simulink model "ColorCodingExample"  (Simulink 7.5)
settings: Solver=FixedStepDiscrete  StartTime=0.0  StopTime=0  FixedStep=0.01  RelTol=1e-3
PostLoadFcn:
  | Workspace_Variable = 1;
InitFcn:
  | ViewValues(1);
undefined symbols (not defined in the file or in its folder): C
libraries: CSA_Library x1
settings Model: Creator=healypa  LastModifiedBy=sufanmi
settings OptimizationCC: InlineInvariantSignals=on  InitFltsAndDblsToZero=on
settings DebuggingCC: SaveWithDisabledLinksMsg=none  SaveWithParameterizedLinksMsg=none  SignalResolutionControl=TryResolveAllWithWarning  MultiTaskDSMMsg=warning  MultiTaskCondExecSysMsg=none  StrictBusMsg=None
settings RTWCC: IncludeERTFirstTime=on
settings GRTTargetCC: TargetFcnLib=ansi_tfl_tmw.mat

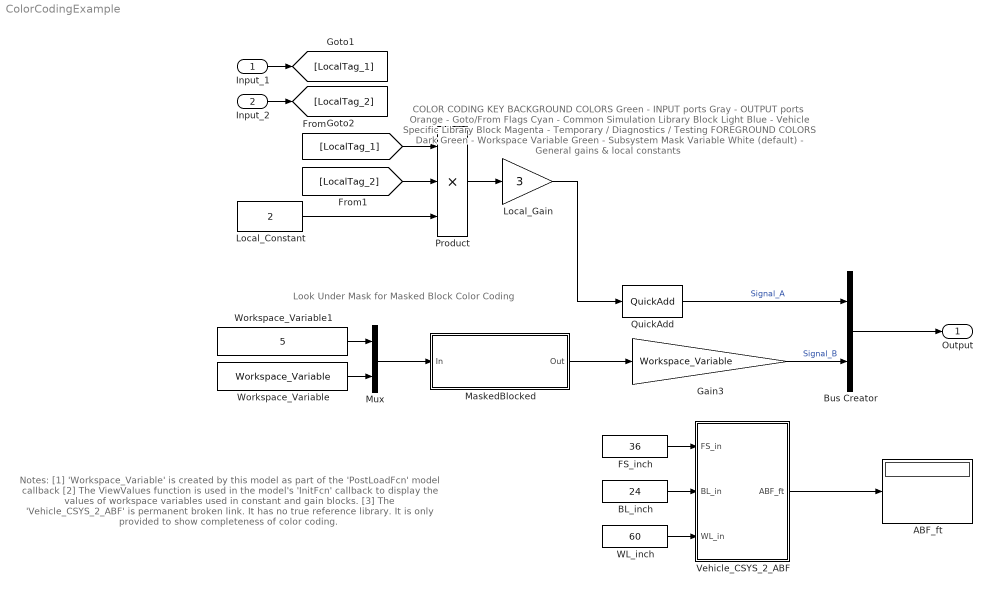
== system ColorCodingExample ==
  note: COLOR CODING KEY
      |
      | BACKGROUND COLORS
      | Green                 - INPUT ports
      | Gray                   - OUTPUT ports
      | Orange               - Goto/From Flags
      | Cyan                   - Common Simulation Library Block
      | Light Blue          - Vehicle Specific Library Block
      | Magenta             - Temporary / Diagnostics / Testing
      |
      | FOREGROUND COLORS
      | Dark Green       - Workspace Variable
      | Green                 - Subsystem Mask Variable
      | White (default) - General gains & local constants
  note: Look Under Mask for
      | Masked Block
      | Color Coding
  note: Notes:
      |
      | [1]  'Workspace_Variable' is created by this
      |        model as part of the 'PostLoadFcn' model callback
      |
      | [2]  The ViewValues function is used in the model's
      |        'InitFcn' callback to display the values of workspace
      |        variables used in constant and gain blocks.
      |
      | [3] The 'Vehicle_CSYS_2_ABF' is permanent broken
      |        link.  It has no true reference library.  It is only
      |        provided to show completeness of color coding.
  Input_1 : Inport  OutDataType=sfix(16)  OutScaling=2^0
  Input_2 : Inport  Port=2  OutDataType=sfix(16)  OutScaling=2^0
  ABF_ft : Display
  BL_inch : Constant  Value=24  OutDataType=sfix(16)  OutScaling=2^0
  Bus Creator : BusCreator  Inputs=2
  FS_inch : Constant  Value=36  OutDataType=sfix(16)  OutScaling=2^0
  Gain3 : Gain  Tag=5  Gain=Workspace_Variable  ParameterDataType=sfix(16)  ParameterScaling=2^0  OutDataType=sfix(16)  OutScaling=2^0
      settings: AttributesFormatString=value: 1
  Local_Constant : Constant  Value=2  OutDataType=sfix(16)  OutScaling=2^0
  Local_Gain : Gain  Gain=3  ParameterDataType=sfix(16)  ParameterScaling=2^0  OutDataType=sfix(16)  OutScaling=2^0
  MaskedBlocked : Subsystem  mask{Mask_Variable=0}
      mask prompts: Mask_Variable "Masked Variable Value"
      mask Display:
      | disp('Masked Block')
      | port_label('input',1,'In');
      | port_label('output',1,'Out');
  Mux : Mux  Inputs=2
  Product : Product  Inputs=3  OutDataType=sfix(16)  OutScaling=2^0  RndMeth=Zero
  QuickAdd : CSA_Library/Utilities/QuickAdd  SystemSampleTime=-1  mskValue=1
  Vehicle_CSYS_2_ABF : Subsystem  AncestorBlock=CSA_Library/Utilities/Vehicle_CSYS_2_ABF
  WL_inch : Constant  Value=60  OutDataType=sfix(16)  OutScaling=2^0
  Workspace_Variable : Constant  Tag=5  Value=Workspace_Variable  OutDataType=sfix(16)  OutScaling=2^0
      settings: AttributesFormatString=value: 1
  Workspace_Variable1 : Constant  Value=5  OutDataType=sfix(16)  OutScaling=2^0
  Output : Outport  OutDataType=sfix(16)  OutScaling=2^0
  wires:
  Input_1/1 -> [LocalTag_1]
  Input_2/1 -> [LocalTag_2]
  [LocalTag_2] -> Product/2
  [LocalTag_1] -> Product/1
  Local_Constant/1 -> Product/3
  Gain3/1 -> Bus Creator/2  "Signal_B"
  Bus Creator/1 -> Output/1
  Product/1 -> Local_Gain/1
  Local_Gain/1 -> QuickAdd/1
  QuickAdd/1 -> Bus Creator/1  "Signal_A"
  MaskedBlocked/1(Out) -> Gain3/1
  FS_inch/1 -> Vehicle_CSYS_2_ABF/1(FS_in)
  BL_inch/1 -> Vehicle_CSYS_2_ABF/2(BL_in)
  WL_inch/1 -> Vehicle_CSYS_2_ABF/3(WL_in)
  Vehicle_CSYS_2_ABF/1(ABF_ft) -> ABF_ft/1
  Mux/1 -> MaskedBlocked/1(In)
  Workspace_Variable1/1 -> Mux/1
  Workspace_Variable/1 -> Mux/2

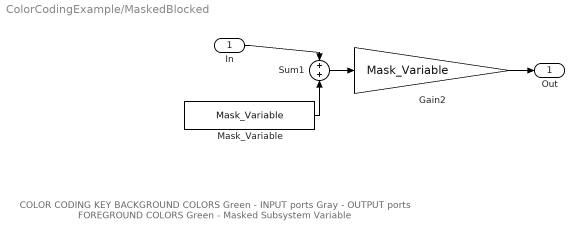
== system ColorCodingExample/MaskedBlocked ==
  note: COLOR CODING KEY
      |
      | BACKGROUND COLORS
      | Green                 - INPUT ports
      | Gray                   - OUTPUT ports
      |
      | FOREGROUND COLORS
      | Green                 - Masked Subsystem Variable
  In : Inport
  Gain2 : Gain  Gain=Mask_Variable  ParameterDataType=sfix(16)  ParameterScaling=2^0  OutDataType=sfix(16)  OutScaling=2^0
  Mask_Variable : Constant  Value=Mask_Variable  OutDataType=sfix(16)  OutScaling=2^0
  Sum1 : Sum  Inputs=+|+  OutDataType=sfix(16)  OutScaling=2^0
  Out : Outport
  wires:
  Mask_Variable/1 -> Sum1/2
  Sum1/1 -> Gain2/1
  In/1 -> Sum1/1
  Gain2/1 -> Out/1

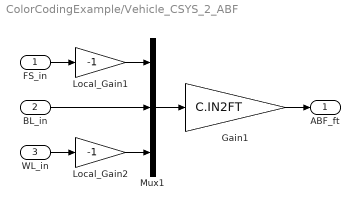
== system ColorCodingExample/Vehicle_CSYS_2_ABF ==
  FS_in : Inport
  BL_in : Inport  Port=2
  WL_in : Inport  Port=3
  Gain1 : Gain  Tag=0.083333  Gain=C.IN2FT  ParameterDataType=sfix(16)  ParameterScaling=2^0  OutDataType=sfix(16)  OutScaling=2^0
      settings: AttributesFormatString=value: 0.083333
  Local_Gain1 : Gain  Gain=-1  ParameterDataType=sfix(16)  ParameterScaling=2^0  OutDataType=sfix(16)  OutScaling=2^0
  Local_Gain2 : Gain  Gain=-1  ParameterDataType=sfix(16)  ParameterScaling=2^0  OutDataType=sfix(16)  OutScaling=2^0
  Mux1 : Mux  Inputs=3
  ABF_ft : Outport
  wires:
  Local_Gain2/1 -> Mux1/3
  Local_Gain1/1 -> Mux1/1
  Mux1/1 -> Gain1/1
  FS_in/1 -> Local_Gain1/1
  Gain1/1 -> ABF_ft/1
  BL_in/1 -> Mux1/2
  WL_in/1 -> Local_Gain2/1
